simulink model "EX2"  (R2023b)
settings: Solver=VariableStepAuto  StartTime=0.0  StopTime=3  RelTol=1e-3
settings Model: Creator=ousso  LastModifiedBy=ousso

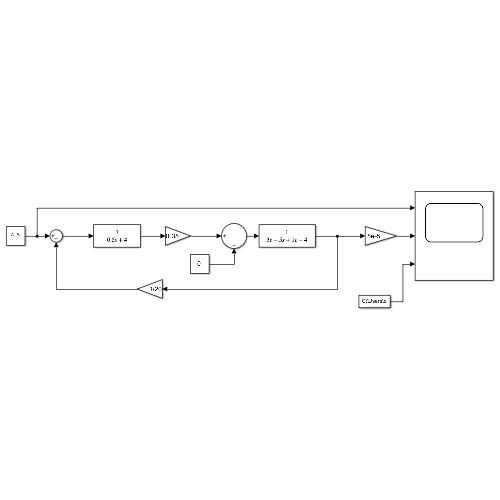
[thumbnail: Simulink's stored preview of the top-level diagram]
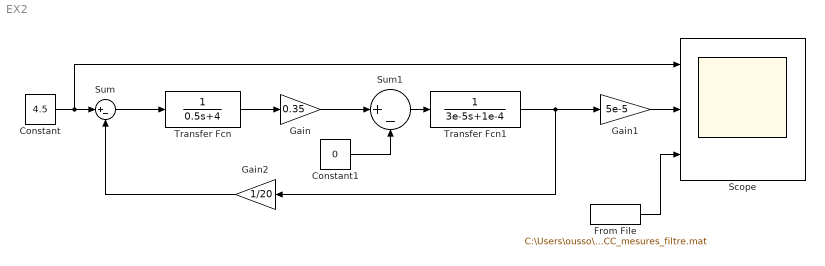
== system EX2 ==
  Constant : Constant  Value=4.5
  Constant1 : Constant  Value=0
  From File : FromFile  FileName=C:\Users\ousso\Desktop\ENIAD\Les Modules\Electronique et Automatique\Automatique\TP\Paramètres_ModèleCausal\MCC_mesures_filtre.mat  SampleTime=0
  Gain : Gain  Gain=0.35
  Gain1 : Gain  Gain=5e-5
  Gain2 : Gain  Gain=1/20
  Scope : Scope  NumInputPorts=3
  Sum : Sum  Inputs=|+-
  Sum1 : Sum  Inputs=|+-
  Transfer Fcn : TransferFcn  Denominator=[0.5 4]
  Transfer Fcn1 : TransferFcn  Denominator=[3e-5 1e-4]
  wires:
  Constant/1 -> Scope/1, Sum/1
  Sum/1 -> Transfer Fcn/1
  Transfer Fcn/1 -> Gain/1
  Gain/1 -> Sum1/1
  Constant1/1 -> Sum1/2
  Sum1/1 -> Transfer Fcn1/1
  Transfer Fcn1/1 -> Gain1/1, Gain2/1
  Gain1/1 -> Scope/2
  Gain2/1 -> Sum/2
  From File/1 -> Scope/3
